simulink model "Park"  (R2022a)
settings: Solver=ode1  StartTime=0.0  StopTime=1  FixedStep=1e-4  RelTol=1e-6  AbsTol=1e-6
PostLoadFcn:
  | , if any(exist('dsrtsu_mdlpostloadfcn', 'file') == [2, 3, 6]), try dsrtsu_mdlpostloadfcn('Execute', bdroot); catch fprintf('Error in PostLoadFcn (dsrtsu_mdlpostloadfcn) for model "%s":\n %s\n', bdroot, lasterr); end, end,
Description:
  | Standard RTI1104 template.
  | Supported MATLAB version:  R2017b.
settings Model: Tag=RTI1104  DSRTSU_INTERNAL_RTI_VER=510  DSRTSU_INTERNAL_RTI_TYPE=rti1104  RTICANMMDATA=struct('GeneralSetupData',struct('modelroot',['C:\Users\habayah\Desktop\TER MERCIER'],'generalsettings',struct('filesettings',struct('destfolder',struct('Name','RTICANMM_FILES','Check',1),'buildfolder',struct('Name','.','Check',1),'AbsDestfolder',struct('Name',['C:\Users\habayah\Desktop\TER MERCIER\RTICANMM_FILES']),'AbsBuildfolder',struct('Name',['C:\Users\habayah\Desktop\TER MERCIER']))),'options',struct('addpaths',1,'rmpaths',1,'addtrcexclusion',logical(1),'cannavigator',struct('checkmonitoring',0),'show_usrtrc',0,'use_usrtrc',0),'advanced',struct('options',[1 1 1 1 1 1 1 1 1 1 1 1 1 1 1 1 1 1 1 1 1 1 1 1 1 1 1 1 1 1 1 1 1 1 1 1 1 1 1 1 1 1 1 1 1 1 1 1 1 1 1 1 1 1 1 1 1 1 1 1 1 1 1 1 1 1 1 1 1 1 1 1 1 1 1 1 1 1 1 1 1 1 1 1 1 1 1 1 1 1 1 1 1 1 1 1 1 1 1 1]),'MPSetup',{{}},'modelname','Park','block','Park'))  DSRTSU_INTERNAL_RTIFLEXRAYCONFIG=110  DSRTSU_INTERNAL_RTIFPGA=110  Creator=habayah  LastModifiedBy=habayah
settings SolverCC: AlgebraicLoopSolver=TrustRegion
settings DataIOCC: ReturnWorkspaceOutputs=off
settings OptimizationCC: BlockReduction=off  OptimizeBlockIOStorage=off  BufferReuse=off  GlobalBufferReuse=off  ExpressionFolding=off  LocalBlockOutputs=off
settings DebuggingCC: UnconnectedInputMsg=warning  UnconnectedOutputMsg=warning  UnconnectedLineMsg=warning  SFMachineParentedDataDiag=warning  ArithmeticOperatorsInVariantConditions=warning
settings HardwareCC: ProdBitPerPointer=32  ProdBitPerSizeT=32  ProdBitPerPtrDiffT=32  ProdLargestAtomicInteger=Integer  ProdEndianess=BigEndian  ProdWordSize=32  ProdHWDeviceType=Custom Processor->Custom  TargetIntDivRoundTo=Zero  TargetEndianess=BigEndian  TargetHWDeviceType=Custom Processor->Custom
settings SFSimCC: SimUseLocalCustomCode=off  MATLABDynamicMemAlloc=off  CustomCodeUndefinedFunction=UseInterfaceOnly
settings RTWCC: Description=dSPACE DS1104 Hardware Platform  SystemTargetFile=rti1104.tlc  MakeCommand=make_rti  TemplateMakefile=rti1104.tmf  RTWUseLocalCustomCode=off
settings CodeAppCC: StateflowObjectComments=on
settings STFCustomTargetCC: MatFileLogging=on  GRTInterface=off  SystemTargetFile=rti1104.tlc
settings GRTTargetCC: TargetLangStandard=C89/C90 (ANSI)  ParMdlRefBuildCompliant=off  CompOptLevelCompliant=off  ConcurrentExecutionCompliant=off  CombineOutputUpdateFcns=off  CPPClassGenCompliant=off  UseToolchainInfoCompliant=off
settings ConfigComp: CovMetricSettings=dswe

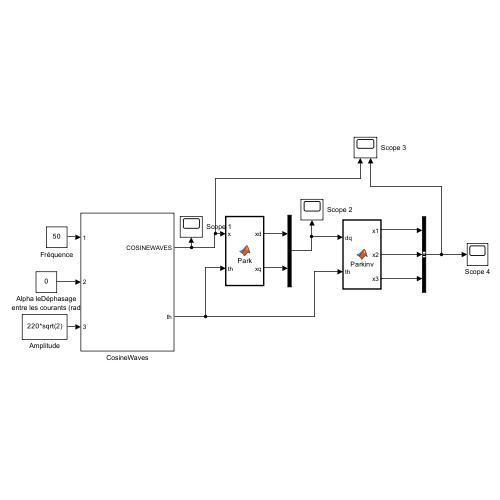
[thumbnail: Simulink's stored preview of the top-level diagram]
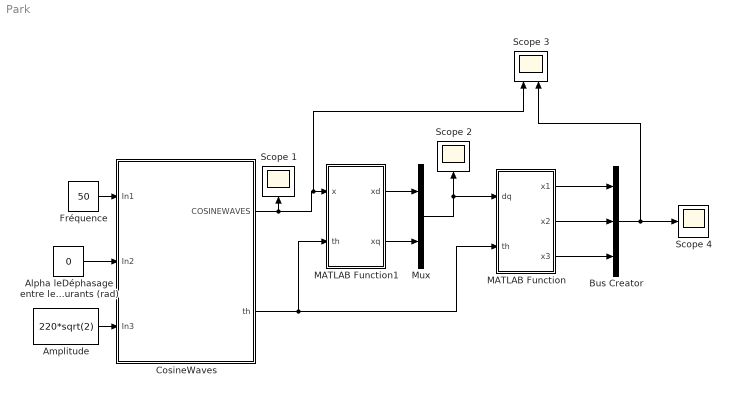
== system Park ==
  Alpha leDéphasage entre les courants (rad) : Constant  Value=0
  Amplitude : Constant  Value=220*sqrt(2)
  Bus Creator : BusCreator  Inputs=3
  CosineWaves : Subsystem
  Fréquence : Constant  Value=50
  MATLAB Function : MATLAB Function  TreatAsAtomicUnit=on
  MATLAB Function1 : MATLAB Function  TreatAsAtomicUnit=on
  Mux : Mux  Inputs=2
  Scope 1 : Scope
  Scope 2 : Scope
  Scope 3 : Scope  NumInputPorts=2
  Scope 4 : Scope
  wires:
  Fréquence/1 -> CosineWaves/1(In1)
  Alpha leDéphasage entre les courants (rad)/1 -> CosineWaves/2(In2)
  CosineWaves/2(th) -> MATLAB Function1/2(th), MATLAB Function/2(th)
  MATLAB Function/1(x1) -> Bus Creator/1
  MATLAB Function/2(x2) -> Bus Creator/2
  MATLAB Function/3(x3) -> Bus Creator/3
  Bus Creator/1 -> Scope 3/2, Scope 4/1
  Mux/1 -> MATLAB Function/1(dq), Scope 2/1
  CosineWaves/1(COSINEWAVES) -> Scope 3/1, MATLAB Function1/1(x), Scope 1/1
  MATLAB Function1/1(xd) -> Mux/1
  MATLAB Function1/2(xq) -> Mux/2
  Amplitude/1 -> CosineWaves/3(In3)

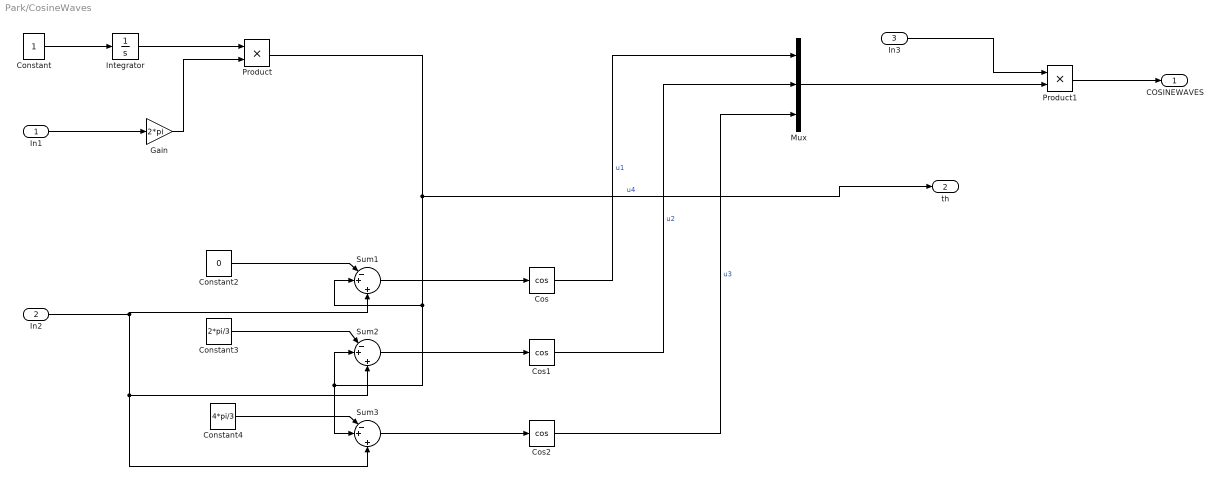
== system Park/CosineWaves ==
  In1 : Inport
  In2 : Inport  Port=2
  In3 : Inport  Port=3
  Constant : Constant
  Constant2 : Constant  Value=0
  Constant3 : Constant  Value=2*pi/3
  Constant4 : Constant  Value=4*pi/3
  Cos : Trigonometry  Operator=cos
  Cos1 : Trigonometry  Operator=cos
  Cos2 : Trigonometry  Operator=cos
  Gain : Gain  Gain=2*pi
  Integrator : Integrator
  Mux : Mux  Inputs=3
  Product : Product
  Product1 : Product
  Sum1 : Sum  Inputs=|-+|+
  Sum2 : Sum  Inputs=|-+|+
  Sum3 : Sum  Inputs=|-+|+
  COSINEWAVES : Outport
  th : Outport  Port=2
  wires:
  Constant/1 -> Integrator/1
  Sum2/1 -> Cos1/1
  In2/1 -> Sum1/3, Sum3/3, Sum2/3
  Product/1 -> th/1, Sum3/2, Sum2/2, Sum1/2  "u4"
  Constant3/1 -> Sum2/1
  Sum3/1 -> Cos2/1
  Sum1/1 -> Cos/1
  Constant2/1 -> Sum1/1
  Constant4/1 -> Sum3/1
  Gain/1 -> Product/2
  Integrator/1 -> Product/1
  In1/1 -> Gain/1
  Cos1/1 -> Mux/2  "u2"
  Cos/1 -> Mux/1  "u1"
  Cos2/1 -> Mux/3  "u3"
  Mux/1 -> Product1/2
  In3/1 -> Product1/1
  Product1/1 -> COSINEWAVES/1

== matlab function Park/MATLAB Function1 ==
  data: x input; xd output; xq output; th input
function [xd,xq] = Park(x,th)
% vd=(2/3)*(u1*cos(th)+u2*cos(th-2*pi/3)+u3*cos(th+2*pi/3));
% vq=(2/3)*(-u1*sin(th)-u2*sin(th-2*pi/3)-u3*sin(th+2*pi/3));
P=(2/3)*[ cos(th) cos(th-2*pi/3) cos(th+2*pi/3);
         -sin(th) -sin(th-2*pi/3) -sin(th+2*pi/3)  ];
prod=P*x;
xd=prod(1);
xq=prod(2);

== matlab function Park/MATLAB Function ==
  data: dq input; x1 output; x2 output; x3 output; th input
function [x1,x2,x3]= Parkinv(dq,th)

parkinv = [ cos(th),           -sin(th); 
          cos(th-2*pi/3), -sin(th-2*pi/3); 
          cos(th+2*pi/3), -sin(th+2*pi/3)];

temp = parkinv * [dq];

x1=temp(1);
x2=temp(2);
x3=temp(3);
